simulink model "cos_toWorkSpace"  (R2015a)
settings: Solver=ode3  StartTime=0.0  StopTime=10  FixedStep=.1  RelTol=1e-3
libraries: simulink x2
settings Model: Creator=ahmed alaa  LastModifiedBy=ahmed alaa

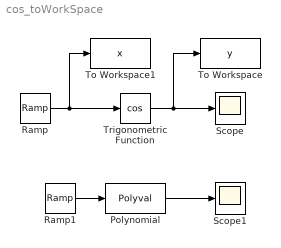
== system cos_toWorkSpace ==
  Polynomial : Polyval  Coefs=[ +2.081618890e-019, -1.441693666e-014, +4.719686976e-010, -8.536869453e-006, +1.621573104e-001, -8.087801117e+001 ]
  Ramp : simulink/Sources/Ramp  slope=1  start=0  X0=0
  Ramp1 : simulink/Sources/Ramp  slope=1  start=0  X0=0
  Scope : Scope
  Scope1 : Scope
  To Workspace : ToWorkspace  VariableName=y  SampleTime=-1
      settings: Save2DSignal=2-D array (concatenate along first dimension)
  To Workspace1 : ToWorkspace  VariableName=x  SampleTime=-1
      settings: Save2DSignal=2-D array (concatenate along first dimension)
  Trigonometric Function : Trigonometry  Operator=cos
  wires:
  Ramp/1 -> Trigonometric Function/1, To Workspace1/1
  Trigonometric Function/1 -> To Workspace/1, Scope/1
  Ramp1/1 -> Polynomial/1
  Polynomial/1 -> Scope1/1
